simulink model "first_cl"  (R2019b)
settings: Solver=VariableStepAuto  StartTime=0.0  StopTime=15  RelTol=1e-3
values from neighbouring files (symbols this model uses):
  K = [66.2259572254 -60.3086645892 5.93307364323 -20.4157003719]    [lqr_K.mat]    (also in lqr_controller.m = lqr(sys,Q,R); swmain.m = lqr_controller(sys2))
  sys = ss(A,B,C,D,-1)    [1b.m]    (also in get_system.m = ss(A,B,C,D); get_system2.m = ss(A,B,C,D); statespace.m = ss(A,B,C,D); swmain.m = get_system(params))
  x_d = desired_state(theta_d, params)    [swmain.m]
undefined symbols (not defined in the file or in its folder): dist
settings Model: Creator=martijndebeuf  LastModifiedBy=Gebruiker

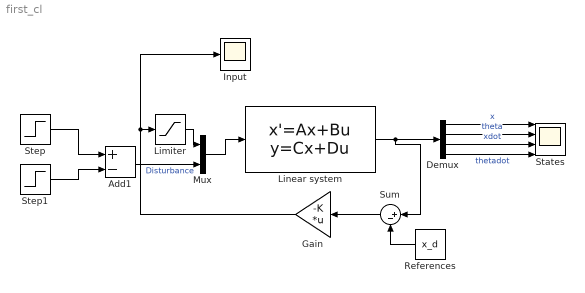
== system first_cl ==
  Add1 : Sum  Inputs=+-
  Demux : Demux
  Gain : Gain  Gain=-K  Multiplication=Matrix(K*u) (u vector)
  Input : Scope
  Limiter : Saturate  UpperLimit=5  LowerLimit=-5
  Linear system : StateSpace  A=sys.A  B=[sys.B,dist]  C=sys.C  D=[sys.D,zeros(4,1)]  InitialCondition=initial_conditions'
  Mux : Mux  Inputs=2
  References : Constant  Value=x_d
  States : Scope  NumInputPorts=4
  Step : Step  Time=8  SampleTime=0
  Step1 : Step  Time=8.1  SampleTime=0
  Sum : Sum  Inputs=|+-
  wires:
  Sum/1 -> Gain/1
  References/1 -> Sum/2
  Demux/1 -> States/1  "x"
  Demux/2 -> States/2  "theta"
  Gain/1 -> Input/1, Limiter/1
  Step/1 -> Add1/1
  Step1/1 -> Add1/2
  Limiter/1 -> Mux/1
  Mux/1 -> Linear system/1
  Add1/1 -> Mux/2  "Disturbance"
  Linear system/1 -> Sum/1, Demux/1
  Demux/3 -> States/3  "xdot"
  Demux/4 -> States/4  "thetadot"
